simulink model "lab2a"  (R2014a)
settings: Solver=FixedStepDiscrete  StartTime=0.0  StopTime=simtime  FixedStep=sampletime  RelTol=1e-3
libraries: dspsrcs4 x3, dspsnks4 x1
settings Model: Creator=micro386  LastModifiedBy=micro386

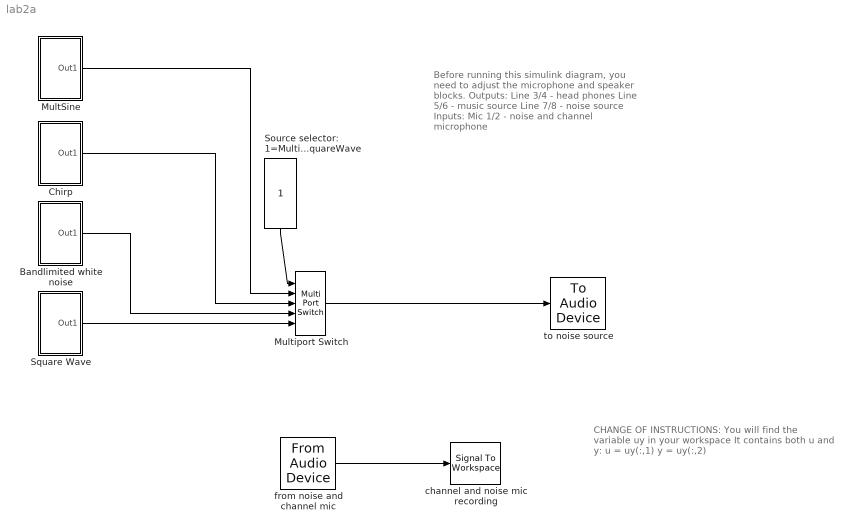
== system lab2a ==
  note: Before running this simulink diagram,
      | you need to adjust the microphone
      | and speaker blocks.
      |
      | Outputs:
      | Line 3/4 - head phones
      | Line 5/6 - music source
      | Line 7/8 - noise source
      |
      | Inputs:
      | Mic 1/2 - noise and channel microphone
  note: CHANGE OF INSTRUCTIONS:
      | You will find the variable uy in your workspace
      |
      | It contains both u and y:
      | u = uy(:,1)
      | y = uy(:,2)
  Bandlimited white noise : Subsystem
  Chirp : Subsystem
  MultSine : Subsystem
  Multiport Switch : MultiPortSwitch  Inputs=4  SaturateOnIntegerOverflow=on  InputSameDT=on
  Source selector: 1=MultiSine 2=Chirp 3=White noise 4=SquareWave : Constant
  Square Wave : Subsystem
  channel and noise mic recording : SignalToWorkspace  VariableName=uy
      settings: CopyFcn=dspblkcopystw(gcbh);
  from noise and channel mic : dspsrcs4/From Audio Device  deviceName=FCA1616 Mic 1/2 (3- Behringer FCA1616 WDM)  numChannels=2  sampleRate=1/sampletime  deviceDatatype=Determine from output data type  autoBufferSize=on  bufferSize=4096  queueDuration=0.1  frameSize=64  outputDatatype=double  defaultInputChannelMapping=on  inputChannelMapping=1:2
  to noise source : dspsnks4/To Audio Device  deviceName=FCA1616 Line 7/8 (3- Behringer FCA1616 WDM)  inheritSampleRate=off  sampleRate=1/sampletime  deviceDatatype=Determine from input data type  autoBufferSize=on  bufferSize=4096  queueDuration=1.0  defaultOutputChannelMapping=on  outputChannelMapping=1:2
  wires:
  Source selector: 1=MultiSine 2=Chirp 3=White noise 4=SquareWave/1 -> Multiport Switch/1
  Chirp/1(Out1) -> Multiport Switch/3
  Square Wave/1(Out1) -> Multiport Switch/5
  Multiport Switch/1 -> to noise source/1
  Bandlimited white noise/1(Out1) -> Multiport Switch/4
  MultSine/1(Out1) -> Multiport Switch/2
  from noise and channel mic/1 -> channel and noise mic recording/1

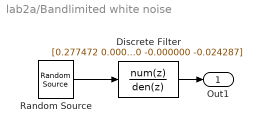
== system lab2a/Bandlimited white noise ==
  Discrete Filter : DiscreteFilter  Numerator=[0.277472 0.000000 -1.387362 0.000000 2.774724 0.000000 -2.774724 0.000000 1.387362 0.000000 -0.277472]*0.3  Denominator=[1.000000 -0.000000 -2.547368 0.000000 2.994845 -0.000000 -1.778046 0.000000 0.534570 -0.000000 -0.024287]  SampleTime=sampletime
  Random Source : dspsrcs4/Random Source  SrcType=Gaussian  NormMethod=Ziggurat  CltLength=12  MinVal=-1  MaxVal=1  MeanVal=0  VarVal=0.6  RepMode=Specify seed  rawSeed=1  IsInherit=off  SampMode=Discrete  SampTime=sampletime  SampFrame=1  DataType=Double  OutComplex=Real
  Out1 : Outport
  wires:
  Discrete Filter/1 -> Out1/1
  Random Source/1 -> Discrete Filter/1

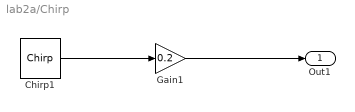
== system lab2a/Chirp ==
  Chirp1 : dspsrcs4/Chirp  sweep=Linear  mode=Bidirectional  f0=600  f1=800  t1=1  Tsweep=10  phase=0  Ts=sampletime  spf=1  datatype=Double
  Gain1 : Gain  Gain=0.2  SaturateOnIntegerOverflow=on  OutDataTypeStr=Inherit: Same as input  ParamDataTypeStr=Inherit: Same as input
  Out1 : Outport
  wires:
  Gain1/1 -> Out1/1
  Chirp1/1 -> Gain1/1

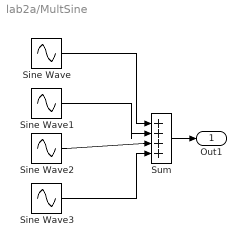
== system lab2a/MultSine ==
  Sine Wave : Sin  Amplitude=.1  Frequency=2*2400  SampleTime=sampletime
  Sine Wave1 : Sin  Amplitude=.1  Frequency=2*3000  SampleTime=sampletime
  Sine Wave2 : Sin  Amplitude=.1  Frequency=2*3600  SampleTime=sampletime
  Sine Wave3 : Sin  Amplitude=.1  Frequency=2*4200  SampleTime=sampletime
  Sum : Sum  Inputs=|++++  SaturateOnIntegerOverflow=on  InputSameDT=on  OutDataTypeStr=Inherit: Same as first input
  Out1 : Outport
  wires:
  Sine Wave/1 -> Sum/1
  Sine Wave1/1 -> Sum/2
  Sine Wave2/1 -> Sum/3
  Sine Wave3/1 -> Sum/4
  Sum/1 -> Out1/1

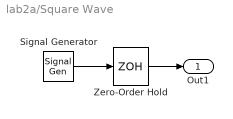
== system lab2a/Square Wave ==
  Signal Generator : SignalGenerator  WaveForm=square  Amplitude=.1  Frequency=100
  Zero-Order Hold : ZeroOrderHold  SampleTime=sampletime
  Out1 : Outport
  wires:
  Zero-Order Hold/1 -> Out1/1
  Signal Generator/1 -> Zero-Order Hold/1
